simulink model "gm_optimised_fil"  (R2024b)
settings: Solver=VariableStepAuto  StartTime=0.0  StopTime=10  RelTol=1e-3
libraries: simulink x1, fillib x1
settings Model: Creator=adubu  LastModifiedBy=adubu
settings OptimizationCC: BlockReduction=off  ConditionallyExecuteInputs=off  DefaultParameterBehavior=Inlined
settings DebuggingCC: AlgebraicLoopMsg=error  InheritedTsInSrcMsg=none
settings HardwareCC: ProdBitPerPointer=32  ProdBitPerSizeT=32  ProdBitPerPtrDiffT=32  ProdLargestAtomicFloat=None  ProdIntDivRoundTo=Undefined  ProdEndianess=Unspecified  ProdWordSize=32  ProdHWDeviceType=ASIC/FPGA->ASIC/FPGA  TargetBitPerPointer=64  TargetBitPerSizeT=64  TargetBitPerPtrDiffT=64  TargetLongLongMode=on  TargetIntDivRoundTo=Zero  TargetEndianess=LittleEndian  TargetWordSize=64  TargetHWDeviceType=Custom Processor->MATLAB Host Computer  ProdEqTarget=off

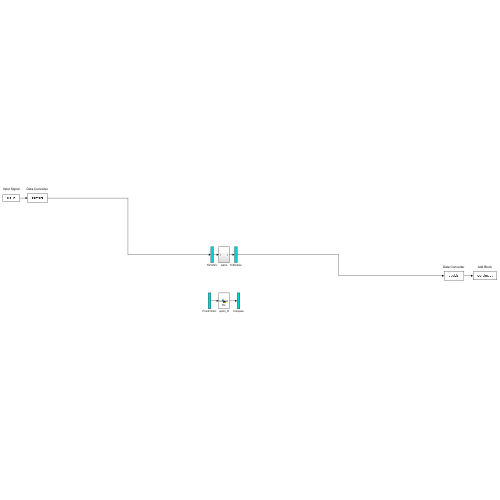
[thumbnail: Simulink's stored preview of the top-level diagram]
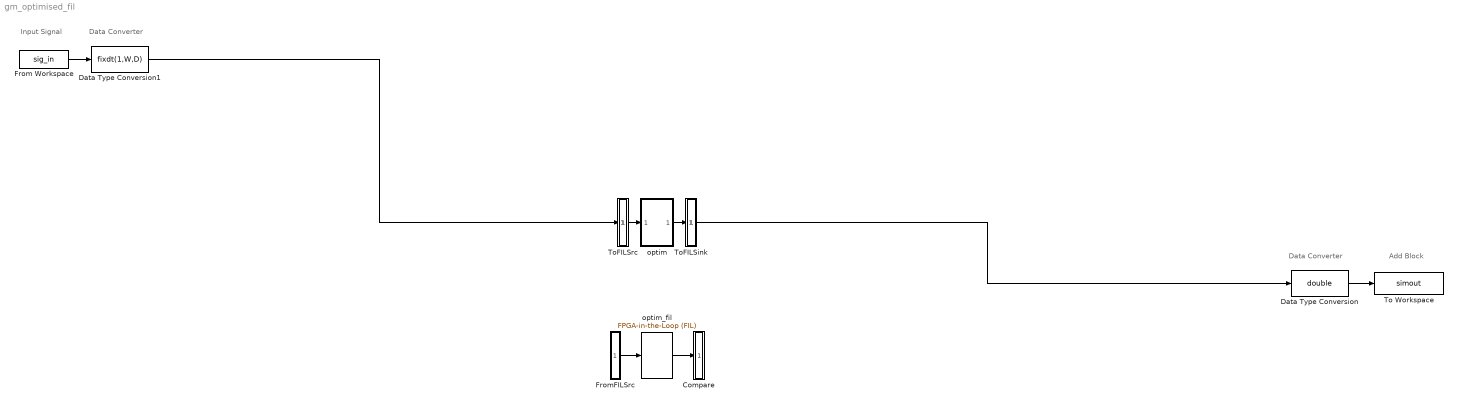
== system gm_optimised_fil ==
  note: Input Signal
  note: Data Converter
  note: Add Block
  note: Data Converter
  Compare : Subsystem
      mask Display: disp('')
  Data Type Conversion : DataTypeConversion  OutDataTypeStr=double  SaturateOnIntegerOverflow=off  RndMeth=Floor
  Data Type Conversion1 : DataTypeConversion  OutDataTypeStr=fixdt(1,W,D)  SaturateOnIntegerOverflow=off  RndMeth=Floor
  From Workspace : FromWorkspace  VariableName=sig_in  SampleTime=1  Interpolate=off  ZeroCross=off  OutputAfterFinalValue=Setting to zero
  FromFILSrc : Subsystem
      mask Display: disp('')
  To Workspace : ToWorkspace  VariableName=simout  SampleTime=-1
  ToFILSink : Subsystem
      mask Display: disp('')
  ToFILSrc : Subsystem
      mask Display: disp('')
  optim : Subsystem
  optim_fil : fillib/FPGA-in-the-Loop (FIL)  ForceInterfaceUpdate=0.90579
  wires:
  Data Type Conversion/1 -> To Workspace/1
  From Workspace/1 -> Data Type Conversion1/1
  ToFILSrc/1(out1) -> optim/1(In1)
  optim/1(Out1) -> ToFILSink/1(in1)
  Data Type Conversion1/1 -> ToFILSrc/1(in1)
  ToFILSink/1(out1) -> Data Type Conversion/1
  FromFILSrc/1(out1) -> optim_fil/1
  optim_fil/1 -> Compare/1(in1)

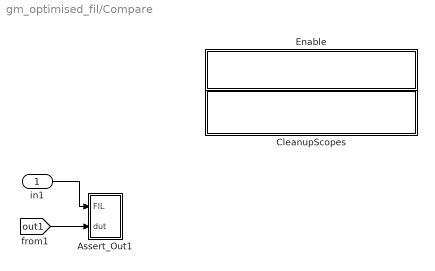
== system gm_optimised_fil/Compare ==
  in1 : Inport
  Assert_Out1 : Subsystem
  CleanupScopes : Subsystem
      settings: OpenFcn=|
      | blkName = gcb; %self block
      | idx = regexp(blkName, '/CleanupScopes$', 'once');
      | blkParent = blkName(1:idx-1);
      | blks=find_system(blkParent, 'LookUnderMasks', 'all','blocktype', 'Scope');
      | for itr = 1:length(blks)
      | 	 hScopeCfg = get_param(blks{itr},'ScopeConfiguration');
      | 	 hScopeCfg.Visible = ~ hScopeCfg.Visible;
      | end
      | drawnow;
      mask Display: fprintf(message('hdlcoder:cosim:vnl_dblclick').getString());
  Enable : Subsystem
      settings: OpenFcn=|
      | blkName = gcb;
      | idx = regexp(blkName, '/Enable$', 'once');
      | blkParent = blkName(1:idx-1);
      | blks=find_system(blkParent, 'LookUnderMasks', 'all','blocktype', 'Assertion');
      | e = get_param(blks{1}, 'Enabled');
      | if strcmp(e, 'on'), f= 'off';, else, f = 'on';, end
      | for ii=1:length(blks), set_param(blks{ii}, 'Enabled', f);, end
      | set_param(gcb, 'MaskDisplay',['fprintf(message(''hdlcoder:cosim:vnl_dblclick_assertions'',','''',upper(e),'''',').getString())']);
      mask Display: fprintf(message('hdlcoder:cosim:vnl_dblclick_assertions','OFF').getString());
  wires:
  in1/1 -> Assert_Out1/1(FIL)
  [out1] -> Assert_Out1/2(dut)

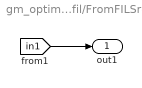
== system gm_optimised_fil/FromFILSrc ==
  out1 : Outport
  wires:
  [in1] -> out1/1

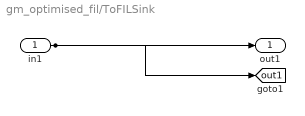
== system gm_optimised_fil/ToFILSink ==
  in1 : Inport
  out1 : Outport
  tag scope: out1=global
  wires:
  in1/1 -> out1/1, [out1]

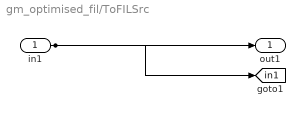
== system gm_optimised_fil/ToFILSrc ==
  in1 : Inport
  out1 : Outport
  tag scope: in1=global
  wires:
  in1/1 -> out1/1, [in1]

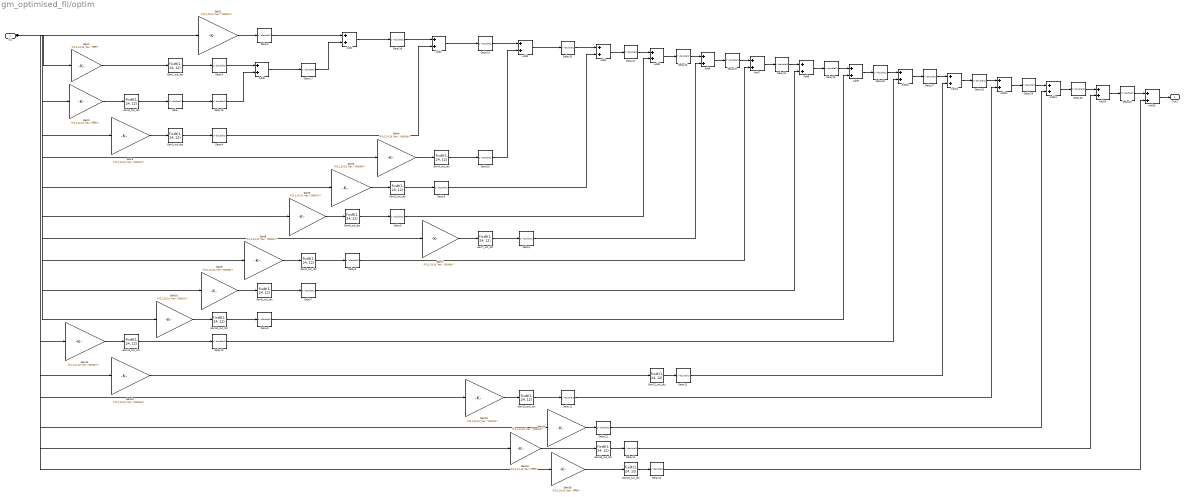
== system gm_optimised_fil/optim ==
  In1 : Inport  OutDataTypeStr=fixdt(1, 24, 12)  PortDimensions=1  SampleTime=1
  Add{0..15} (16 alike) : Sum  OutDataTypeStr=fixdt(1, 24, 12)  AccumDataTypeStr=fixdt(1, 24, 12)  SampleTime=1
  Delay{,1..32} (33 alike) : Delay  DelayLength=double(1)  InitialCondition=0  SampleTime=1
  Gain0 : Gain  Gain="fi(0,1,24,10,\"hex\",\"fffffe\")"  ParamDataTypeStr=fixdt(1, 24, 10)  OutDataTypeStr=fixdt(1, 48, 22)  SampleTime=1
  Gain0_out_dtc : DataTypeConversion  OutDataTypeStr=fixdt(1, 24, 12)  SampleTime=1  SaturateOnIntegerOverflow=off  RndMeth=Floor
  Gain1 : Gain  Gain="fi(0,1,24,10,\"hex\",\"ffffff\")"  ParamDataTypeStr=fixdt(1, 24, 10)  OutDataTypeStr=fixdt(1, 48, 22)  SampleTime=1
  Gain10 : Gain  Gain="fi(0,1,24,10,\"hex\",\"00007c\")"  ParamDataTypeStr=fixdt(1, 24, 10)  OutDataTypeStr=fixdt(1, 48, 22)  SampleTime=1
  Gain10_out_dtc : DataTypeConversion  OutDataTypeStr=fixdt(1, 24, 12)  SampleTime=1  SaturateOnIntegerOverflow=off  RndMeth=Floor
  Gain11 : Gain  Gain="fi(0,1,24,10,\"hex\",\"000054\")"  ParamDataTypeStr=fixdt(1, 24, 10)  OutDataTypeStr=fixdt(1, 48, 22)  SampleTime=1
  Gain11_out_dtc : DataTypeConversion  OutDataTypeStr=fixdt(1, 24, 12)  SampleTime=1  SaturateOnIntegerOverflow=off  RndMeth=Floor
  Gain12 : Gain  Gain="fi(0,1,24,10,\"hex\",\"00002e\")"  ParamDataTypeStr=fixdt(1, 24, 10)  OutDataTypeStr=fixdt(1, 48, 22)  SampleTime=1
  Gain12_out_dtc : DataTypeConversion  OutDataTypeStr=fixdt(1, 24, 12)  SampleTime=1  SaturateOnIntegerOverflow=off  RndMeth=Floor
  Gain13 : Gain  Gain="fi(0,1,24,10,\"hex\",\"000012\")"  ParamDataTypeStr=fixdt(1, 24, 10)  OutDataTypeStr=fixdt(1, 48, 22)  SampleTime=1
  Gain13_out_dtc : DataTypeConversion  OutDataTypeStr=fixdt(1, 24, 12)  SampleTime=1  SaturateOnIntegerOverflow=off  RndMeth=Floor
  Gain14 : Gain  Gain="fi(0,1,24,10,\"hex\",\"000004\")"  ParamDataTypeStr=fixdt(1, 24, 10)  OutDataTypeStr=fixdt(1, 24, 12)  SampleTime=1
  Gain15 : Gain  Gain="fi(0,1,24,10,\"hex\",\"ffffff\")"  ParamDataTypeStr=fixdt(1, 24, 10)  OutDataTypeStr=fixdt(1, 48, 22)  SampleTime=1
  Gain15_out_dtc : DataTypeConversion  OutDataTypeStr=fixdt(1, 24, 12)  SampleTime=1  SaturateOnIntegerOverflow=off  RndMeth=Floor
  Gain16 : Gain  Gain="fi(0,1,24,10,\"hex\",\"fffffe\")"  ParamDataTypeStr=fixdt(1, 24, 10)  OutDataTypeStr=fixdt(1, 48, 22)  SampleTime=1
  Gain16_out_dtc : DataTypeConversion  OutDataTypeStr=fixdt(1, 24, 12)  SampleTime=1  SaturateOnIntegerOverflow=off  RndMeth=Floor
  Gain1_out_dtc : DataTypeConversion  OutDataTypeStr=fixdt(1, 24, 12)  SampleTime=1  SaturateOnIntegerOverflow=off  RndMeth=Floor
  Gain2 : Gain  Gain="fi(0,1,24,10,\"hex\",\"000004\")"  ParamDataTypeStr=fixdt(1, 24, 10)  OutDataTypeStr=fixdt(1, 24, 12)  SampleTime=1
  Gain3 : Gain  Gain="fi(0,1,24,10,\"hex\",\"000012\")"  ParamDataTypeStr=fixdt(1, 24, 10)  OutDataTypeStr=fixdt(1, 48, 22)  SampleTime=1
  Gain3_out_dtc : DataTypeConversion  OutDataTypeStr=fixdt(1, 24, 12)  SampleTime=1  SaturateOnIntegerOverflow=off  RndMeth=Floor
  Gain4 : Gain  Gain="fi(0,1,24,10,\"hex\",\"00002e\")"  ParamDataTypeStr=fixdt(1, 24, 10)  OutDataTypeStr=fixdt(1, 48, 22)  SampleTime=1
  Gain4_out_dtc : DataTypeConversion  OutDataTypeStr=fixdt(1, 24, 12)  SampleTime=1  SaturateOnIntegerOverflow=off  RndMeth=Floor
  Gain5 : Gain  Gain="fi(0,1,24,10,\"hex\",\"000054\")"  ParamDataTypeStr=fixdt(1, 24, 10)  OutDataTypeStr=fixdt(1, 48, 22)  SampleTime=1
  Gain5_out_dtc : DataTypeConversion  OutDataTypeStr=fixdt(1, 24, 12)  SampleTime=1  SaturateOnIntegerOverflow=off  RndMeth=Floor
  Gain6 : Gain  Gain="fi(0,1,24,10,\"hex\",\"00007c\")"  ParamDataTypeStr=fixdt(1, 24, 10)  OutDataTypeStr=fixdt(1, 48, 22)  SampleTime=1
  Gain6_out_dtc : DataTypeConversion  OutDataTypeStr=fixdt(1, 24, 12)  SampleTime=1  SaturateOnIntegerOverflow=off  RndMeth=Floor
  Gain7 : Gain  Gain="fi(0,1,24,10,\"hex\",\"00009c\")"  ParamDataTypeStr=fixdt(1, 24, 10)  OutDataTypeStr=fixdt(1, 48, 22)  SampleTime=1
  Gain7_out_dtc : DataTypeConversion  OutDataTypeStr=fixdt(1, 24, 12)  SampleTime=1  SaturateOnIntegerOverflow=off  RndMeth=Floor
  Gain8 : Gain  Gain="fi(0,1,24,10,\"hex\",\"0000a7\")"  ParamDataTypeStr=fixdt(1, 24, 10)  OutDataTypeStr=fixdt(1, 48, 22)  SampleTime=1
  Gain8_out_dtc : DataTypeConversion  OutDataTypeStr=fixdt(1, 24, 12)  SampleTime=1  SaturateOnIntegerOverflow=off  RndMeth=Floor
  Gain9 : Gain  Gain="fi(0,1,24,10,\"hex\",\"00009c\")"  ParamDataTypeStr=fixdt(1, 24, 10)  OutDataTypeStr=fixdt(1, 48, 22)  SampleTime=1
  Gain9_out_dtc : DataTypeConversion  OutDataTypeStr=fixdt(1, 24, 12)  SampleTime=1  SaturateOnIntegerOverflow=off  RndMeth=Floor
  Out1 : Outport  SampleTime=1
  wires:
  Add15/1 -> Out1/1
  Delay32/1 -> Add15/1
  Add14/1 -> Delay32/1
  Delay30/1 -> Add14/1
  Add13/1 -> Delay30/1
  Delay29/1 -> Add13/1
  Add12/1 -> Delay29/1
  Delay28/1 -> Add12/1
  Add11/1 -> Delay28/1
  Delay27/1 -> Add11/1
  Add10/1 -> Delay27/1
  Delay26/1 -> Add10/1
  Add9/1 -> Delay26/1
  Delay25/1 -> Add9/1
  Add8/1 -> Delay25/1
  Delay24/1 -> Add8/1
  Add7/1 -> Delay24/1
  Delay23/1 -> Add7/1
  Delay31/1 -> Add15/2
  Gain12_out_dtc/1 -> Delay11/1
  Add5/1 -> Delay22/1
  Gain16_out_dtc/1 -> Delay31/1
  Delay14/1 -> Add14/2
  Gain15_out_dtc/1 -> Delay14/1
  Add4/1 -> Delay21/1
  Gain14/1 -> Delay13/1
  Delay20/1 -> Add4/1
  Gain15/1 -> Gain15_out_dtc/1
  Delay22/1 -> Add6/1
  Gain13_out_dtc/1 -> Delay12/1
  Gain13/1 -> Gain13_out_dtc/1
  Gain7_out_dtc/1 -> Delay1/1
  Gain4_out_dtc/1 -> Delay15/1
  Delay9/1 -> Add5/2
  Gain5_out_dtc/1 -> Delay6/1
  Delay11/1 -> Add11/2
  Gain4/1 -> Gain4_out_dtc/1
  Delay18/1 -> Add2/1
  Delay5/1 -> Add7/2
  Gain6_out_dtc/1 -> Delay9/1
  Add2/1 -> Delay19/1
  Gain5/1 -> Gain5_out_dtc/1
  Add6/1 -> Delay23/1
  Add1/1 -> Delay18/1
  Delay7/1 -> Add8/2
  Delay13/1 -> Add13/2
  Gain8_out_dtc/1 -> Delay5/1
  Gain6/1 -> Gain6_out_dtc/1
  Delay8/1 -> Add9/2
  Gain9_out_dtc/1 -> Delay7/1
  Delay15/1 -> Add3/2
  Gain8/1 -> Gain8_out_dtc/1
  Delay10/1 -> Add10/2
  Add3/1 -> Delay20/1
  Gain16/1 -> Gain16_out_dtc/1
  Gain10_out_dtc/1 -> Delay8/1
  Delay19/1 -> Add3/1
  Gain9/1 -> Gain9_out_dtc/1
  Delay4/1 -> Add2/2
  Delay12/1 -> Add12/2
  Delay16/1 -> Add0/2
  Gain7/1 -> Gain7_out_dtc/1
  Delay3/1 -> Add0/1
  Gain2/1 -> Delay2/1
  Gain10/1 -> Gain10_out_dtc/1
  Delay2/1 -> Add1/1
  Gain3_out_dtc/1 -> Delay4/1
  Delay1/1 -> Add6/2
  Delay/1 -> Delay16/1
  Gain1_out_dtc/1 -> Delay3/1
  Gain3/1 -> Gain3_out_dtc/1
  Gain11/1 -> Gain11_out_dtc/1
  Gain0/1 -> Gain0_out_dtc/1
  Gain1/1 -> Gain1_out_dtc/1
  Delay17/1 -> Add1/2
  Gain0_out_dtc/1 -> Delay/1
  In1/1 -> Gain11/1, Gain0/1, Gain1/1, Gain6/1, Gain12/1, Gain10/1, Gain13/1, Gain16/1, Gain14/1, Gain15/1, Gain2/1, Gain3/1, Gain4/1, Gain5/1, Gain7/1, Gain8/1, Gain9/1
  Add0/1 -> Delay17/1
  Delay6/1 -> Add4/2
  Gain11_out_dtc/1 -> Delay10/1
  Delay21/1 -> Add5/1
  Gain12/1 -> Gain12_out_dtc/1

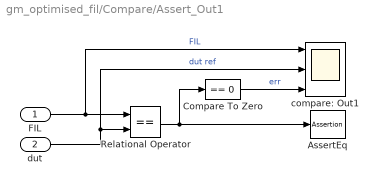
== system gm_optimised_fil/Compare/Assert_Out1 ==
  FIL : Inport
  dut : Inport  Port=2
  AssertEq : Assertion  StopWhenAssertionFail=off
  Compare To Zero : simulink/Logic and Bit Operations/Compare To Zero  relop===  OutDataTypeStr=boolean
  Relational Operator : RelationalOperator  Operator===  OutDataTypeStr=boolean  InputSameDT=off
  compare: Out1 : Scope  NumInputPorts=3
  wires:
  Compare To Zero/1 -> compare: Out1/3  "err"
  Relational Operator/1 -> Compare To Zero/1, AssertEq/1
  FIL/1 -> compare: Out1/1, Relational Operator/1  "FIL"
  dut/1 -> compare: Out1/2, Relational Operator/2  "dut ref"

== system gm_optimised_fil/Compare/CleanupScopes ==

== system gm_optimised_fil/Compare/Enable ==
